simulink model "motor_speed_reference"  (R2020b)
settings: Solver=FixedStepDiscrete  StartTime=0.0  StopTime=10.0  FixedStep=double(Ts)  RelTol=1e-3
undefined symbols (not defined in the file): ReductionGearRaio, TireRadius
settings Model: DataDictionary=motor_speed_reference.sldd  Creator=Dmitry  LastModifiedBy=Dmitry

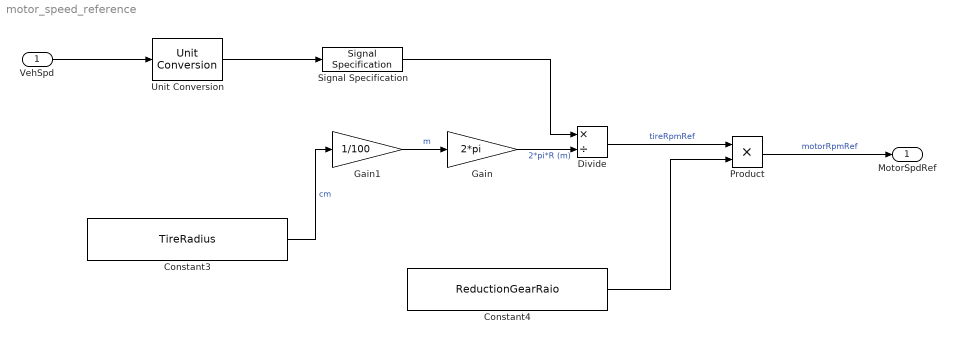
== system motor_speed_reference ==
  VehSpd : Inport  Unit=km/hr
  Constant3 : Constant  Value=TireRadius
  Constant4 : Constant  Value=ReductionGearRaio
  Divide : Product  Inputs=*/
  Gain : Gain  Gain=2*pi
  Gain1 : Gain  Gain=1/100
  Product : Product
  Signal Specification : SignalSpecification  Unit=m/min
  Unit Conversion : UnitConversion
  MotorSpdRef : Outport  Unit=rpm  VectorParamsAs1DForOutWhenUnconnected=off
  wires:
  VehSpd/1 -> Unit Conversion/1
  Constant3/1 -> Gain1/1  "cm"
  Gain1/1 -> Gain/1  "m"
  Unit Conversion/1 -> Signal Specification/1
  Product/1 -> MotorSpdRef/1  "motorRpmRef"
  Gain/1 -> Divide/2  "2*pi*R (m)"
  Divide/1 -> Product/1  "tireRpmRef"
  Constant4/1 -> Product/2
  Signal Specification/1 -> Divide/1
